simulink model "RPM_test"  (R2024a)
settings: Solver=FixedStepAuto  StartTime=0.0  StopTime=6  FixedStep=1e-5  RelTol=1e-3
values from neighbouring files (symbols this model uses):
  B = 0.002277    [initial_value.m]
  J = 0.00782    [initial_value.m]
  Lambda_m = 0.30175    [initial_value.m]
  Ld = 18e-3    (= 0.018)    [initial_value.m]
  Ldq = Ld - Lq    [inital.m]
  Lq = 32e-3    (= 0.032)    [initial_value.m]
  Polepairs = 3    [initial_value.m]
  Rs = 2.5    [initial_value.m]
  timestep = 1e-5    (= 1e-05)    [inital.m]
  V = [V_11 V_12;V_21 V_22]    [Create_MVG.m]
undefined symbols (not defined in the file or in its folder): sigbuilder_block
libraries: spsControlledVoltageSourceLib x3, spsPermanentMagnetSynchronousMachineLib x1, spsGroundLib x1, sps_lib x1
settings Model: Creator=User  LastModifiedBy=User

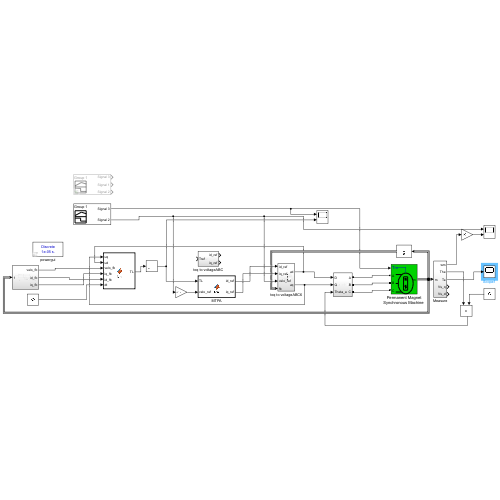
[thumbnail: Simulink's stored preview of the top-level diagram]
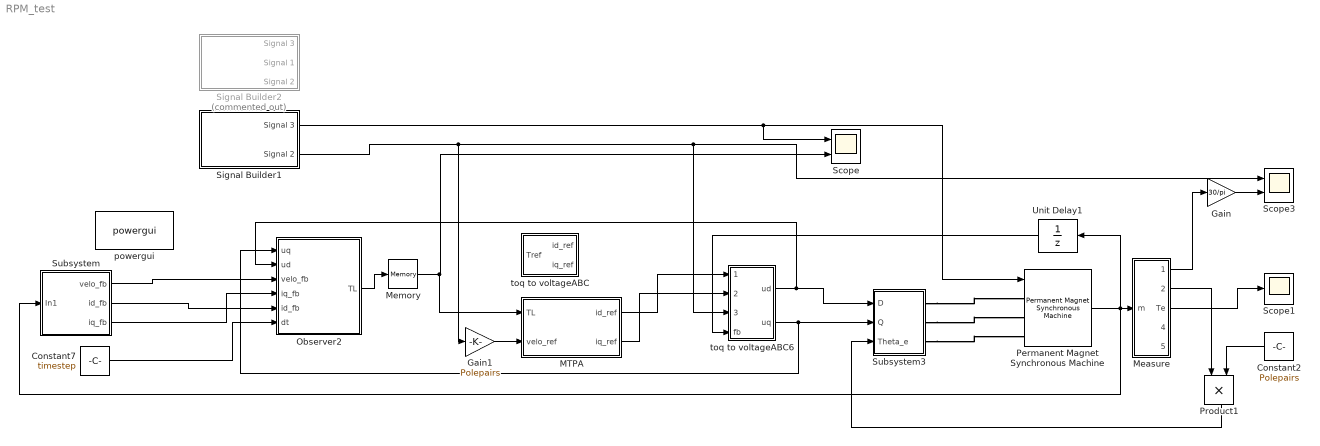
== system RPM_test ==
  Constant2 : Constant  Value=Polepairs
  Constant7 : Constant  Value=timestep
  Gain : Gain  Gain=30/pi
  Gain1 : Gain  Gain=Polepairs
  MTPA : MATLAB Function  TreatAsAtomicUnit=on
  Measure : Subsystem
  Memory : Memory
  Observer2 : MATLAB Function  TreatAsAtomicUnit=on
  "Permanent Magnet Synchronous Machine " : spsPermanentMagnetSynchronousMachineLib/Permanent Magnet Synchronous Machine  NbPhases=3  FluxDistribution=Sinusoidal  RotorType=Salient-pole  MechanicalLoad=Torque Tm  PresetModel=No  ShowDetailedParameters=on  MeasurementBus=off  Resistance=Rs  Inductance=8.5e-3  dqInductances=[Ld Lq]  La=5.7e-3  MachineConstant=Flux linkage established by magnets (V.s)  Flux=Lambda_m  VoltageCst=14.8877  TorqueCst=0.12312  Flat=120  Mechanical=[J B Polepairs]  PolePairs=4  InitialConditions=[0,0, 0,0]  InitialConditions5ph=[0 0 0 0 0 0]  RefAngle=Aligned with phase A axis (original Park)  IterativeDiscreteModel=Trapezoidal non iterative  TsBlock=-1  TsPowergui=0
  Product1 : Product
  Scope : Scope  NumInputPorts=2
  Scope1 : Scope
  Scope3 : Scope  NumInputPorts=2
  Signal Builder1 : Subsystem  Tag=STV Subsys  LoadFcn=sigbuilder_block('load');  StartFcn=sigbuilder_block('start');  StopFcn=sigbuilder_block('stop');  ClipboardFcn=sigbuilder_block('clipboard');  mask(Sigbuilder block){tuvar=[0:10]}
      mask help: Simulink:masks:SigbuilderBlock_MD
      mask init:
      | if ~strcmp(get_param(bdroot(gcbh),'SimulationStatus'),'stopped') tuvar = sigbuilder_block('maskInit'); end
      settings: CopyFcn=sigbuilder_block('copy');  DeleteFcn=sigbuilder_block('delete');  ModelCloseFcn=sigbuilder_block('modelClose');  PreSaveFcn=sigbuilder_block('preSave');  PauseFcn=sigbuilder_block('pause');  ContinueFcn=sigbuilder_block('continue');  NameChangeFcn=sigbuilder_block('namechange');  OpenFcn=sigbuilder_block('open',[524.25 120.75 551.25 399.75 ]);  CloseFcn=sigbuilder_block('close');
      mask Display: plot(0, 0, 100, 100,[2, 2, 32, 32, 2], [68, 8, 8, 68, 68],[32, 2], [38, 38], [32, 19, 2],[53, 60, 44], [32, 17, 17, 2],[16, 16, 31, 31]);txt = getActiveGroup(gcbh);text(2, 100, txt,'verticalAlignment', 'top');
  Signal Builder2 : Subsystem  Tag=STV Subsys  Commented=on  LoadFcn=sigbuilder_block('load');  StartFcn=sigbuilder_block('start');  StopFcn=sigbuilder_block('stop');  ClipboardFcn=sigbuilder_block('clipboard');  mask(Sigbuilder block){tuvar=[0:10]}
      mask help: Simulink:masks:SigbuilderBlock_MD
      mask init:
      | if ~strcmp(get_param(bdroot(gcbh),'SimulationStatus'),'stopped') tuvar = sigbuilder_block('maskInit'); end
      settings: CopyFcn=sigbuilder_block('copy');  DeleteFcn=sigbuilder_block('delete');  ModelCloseFcn=sigbuilder_block('modelClose');  PreSaveFcn=sigbuilder_block('preSave');  PauseFcn=sigbuilder_block('pause');  ContinueFcn=sigbuilder_block('continue');  NameChangeFcn=sigbuilder_block('namechange');  OpenFcn=sigbuilder_block('open',[524.25 120.75 551.25 399.75 ]);  CloseFcn=sigbuilder_block('close');
      mask Display: plot(0, 0, 100, 100,[2, 2, 32, 32, 2], [68, 8, 8, 68, 68],[32, 2], [38, 38], [32, 19, 2],[53, 60, 44], [32, 17, 17, 2],[16, 16, 31, 31]);txt = getActiveGroup(gcbh);text(2, 100, txt,'verticalAlignment', 'top');
  Subsystem : Subsystem
  Subsystem3 : Subsystem
  Unit Delay1 : UnitDelay  SampleTime=1e-5  HasFrameUpgradeWarning=on
  powergui : sps_lib/powergui  Priority=1  SimulationMode=Discrete  SampleTime=timestep  frequency=60  Iterations=50  frequencyindice=0  Pbase=100e6  ErrMax=1e-4  UnitsV=kV  UnitsW=MW  buscounter=0  FunctionMessages=off  echomessages=off  EnableUseOfTLC=off  CurrentSourceSwitches=off  DisableSnubberDevices=off  DisableRonSwitches=off  DisableVfSwitches=off  DisplayEquations=off  AutomaticDiscreteSolvers=off  SolverType=Tustin/Backward Euler (TBE)  Interpol=off  ExternalGateDelay=off  methode=off  Ts=100  x0status=blocks  SPID=on  SwTol=0  HookPort=off  NonlinearTolerance=1e-4  nMaxIteration=100  ContinueOnMaxIteration=off  RestoreLinks=warning  ResistiveCurrentMeasurement=off  Frange=[0:2:500]  Ylog=off  Xlog=on  ShowGrid=off  save=off  variable=ZData  structure=0  ZoomFFT=off  StartTime=0.0  cycles=1  DisplayStyle=1  fundamental=60  FreqAxis=off  MaxFrequency=1000  frequencyindicesteady=1  RmsSteady=1  display=off
  toq to voltageABC : Subsystem
  toq to voltageABC6 : Subsystem
  wires:
  "Permanent Magnet Synchronous Machine "/1 -> Unit Delay1/1, Measure/1(m), Subsystem/1(In1)
  Constant2/1 -> Product1/2
  Measure/2(The) -> Product1/1
  Unit Delay1/1 -> toq to voltageABC6/4(fb)
  toq to voltageABC6/1(ud) -> Observer2/2(ud), Subsystem3/1(D)
  toq to voltageABC6/2(uq) -> Observer2/1(uq), Subsystem3/2(Q)
  Product1/1 -> Subsystem3/3(Theta_e)
  Subsystem/1(velo_fb) -> Observer2/3(velo_fb)
  Subsystem/2(id_fb) -> Observer2/5(id_fb)
  Subsystem/3(iq_fb) -> Observer2/4(iq_fb)
  Signal Builder1/2(Signal 2) -> Gain1/1, toq to voltageABC6/3(velo_ref), Scope3/1
  Observer2/1(TL) -> Memory/1
  Constant7/1 -> Observer2/6(dt)
  Measure/1(wm) -> Gain/1
  Gain/1 -> Scope3/2
  Signal Builder1/1(Signal 3) -> "Permanent Magnet Synchronous Machine "/1, Scope/1
  Gain1/1 -> MTPA/2(velo_ref)
  Memory/1 -> MTPA/1(TL), Scope/2
  Measure/3(Te) -> Scope1/1
  MTPA/1(id_ref) -> toq to voltageABC6/1(id_ref)
  MTPA/2(iq_ref) -> toq to voltageABC6/2(iq_ref)
  connections:
  Subsystem3/RConn1 -- "Permanent Magnet Synchronous Machine "/LConn1
  Subsystem3/RConn2 -- "Permanent Magnet Synchronous Machine "/LConn2
  Subsystem3/RConn3 -- "Permanent Magnet Synchronous Machine "/LConn3

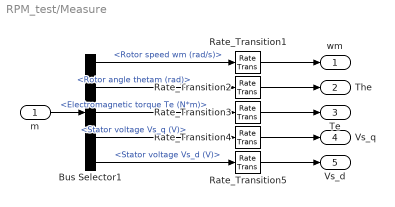
== system RPM_test/Measure ==
  m : Inport
  Bus Selector1 : BusSelector  OutputSignals=Rotor speed wm (rad/s),Rotor angle thetam (rad),Electromagnetic torque Te (N*m),Stator voltage Vs_q (V),Stator voltage Vs_d (V)
  Rate_Transition{1..5} (5 alike) : RateTransition  Integrity=off
  wm : Outport
  The : Outport  Port=2
  Te : Outport  Port=3
  Vs_q : Outport  Port=4
  Vs_d : Outport  Port=5
  wires:
  Bus Selector1/5 -> Rate_Transition5/1  "<Stator voltage Vs_d (V)>"
  Bus Selector1/4 -> Rate_Transition4/1  "<Stator voltage Vs_q (V)>"
  Bus Selector1/1 -> Rate_Transition1/1  "<Rotor speed wm (rad/s)>"
  m/1 -> Bus Selector1/1
  Bus Selector1/3 -> Rate_Transition3/1  "<Electromagnetic torque Te (N*m)>"
  Bus Selector1/2 -> Rate_Transition2/1  "<Rotor angle thetam (rad)>"
  Rate_Transition1/1 -> wm/1
  Rate_Transition2/1 -> The/1
  Rate_Transition3/1 -> Te/1
  Rate_Transition4/1 -> Vs_q/1
  Rate_Transition5/1 -> Vs_d/1

== system RPM_test/Signal Builder1 ==
  Demux : Demux  Tag=STV Demux  Outputs=2
      settings: DisplayOption=none
  FromWs : FromWorkspace  Tag=STV FromWs  VariableName=tuvar
      SigBuilderData=|
      | common.afterFinalStr = 'Extrapolate'
      | common.sampleTime = 0
      | dataSet.timeRange = [0 6]
      | dataSet.name = 'Group 1'
      | sbobj.Groups.Name = 'Group 1'
      | sbobj.Groups.Signals(1).Name = 'Signal 3'
      | sbobj.Groups.Signals(1).XData = [0 2 3 4 5 6]
      | sbobj.Groups.Signals(1).YData = [0 0 1 1 0 0]
      | sbobj.Groups.Signals(2).Name = 'Signal 2'
      | sbobj.Groups.Signals(2).XData = [0 2 3 6]
      | sbobj.Groups.Signals(2).YData = [0 10 10 10]
      | sbobj.Groups.TimeRange = [0 6]
  Signal 3 : Outport  Tag=STV Outport
  Signal 2 : Outport  Tag=STV Outport  Port=2
  wires:
  FromWs/1 -> Demux/1
  Demux/1 -> Signal 3/1
  Demux/2 -> Signal 2/1

== system RPM_test/Signal Builder2 ==
  Demux : Demux  Tag=STV Demux  Outputs=3
      settings: DisplayOption=none
  FromWs : FromWorkspace  Tag=STV FromWs  VariableName=tuvar
      SigBuilderData=|
      | common.afterFinalStr = 'Extrapolate'
      | common.sampleTime = 0
      | dataSet.timeRange = [0 6]
      | dataSet.name = 'Group 1'
      | sbobj.Groups.Name = 'Group 1'
      | sbobj.Groups.Signals(1).Name = 'Signal 3'
      | sbobj.Groups.Signals(1).XData = [0 6]
      | sbobj.Groups.Signals(1).YData = [1 1]
      | sbobj.Groups.Signals(2).Name = 'Signal 1'
      | sbobj.Groups.Signals(2).XData = [0 2 4 6]
      | sbobj.Groups.Signals(2).YData = [0 1.5 1.5 0]
      | sbobj.Groups.Signals(3).Name = 'Signal 2'
      | sbobj.Groups.Signals(3).XData = [0 6]
      | sbobj.Groups.Signals(3).YData = [0 10]
      | sbobj.Groups.TimeRange = [0 6]
  Signal 3 : Outport  Tag=STV Outport
  Signal 1 : Outport  Tag=STV Outport  Port=2
  Signal 2 : Outport  Tag=STV Outport  Port=3
  wires:
  FromWs/1 -> Demux/1
  Demux/1 -> Signal 3/1
  Demux/2 -> Signal 1/1
  Demux/3 -> Signal 2/1

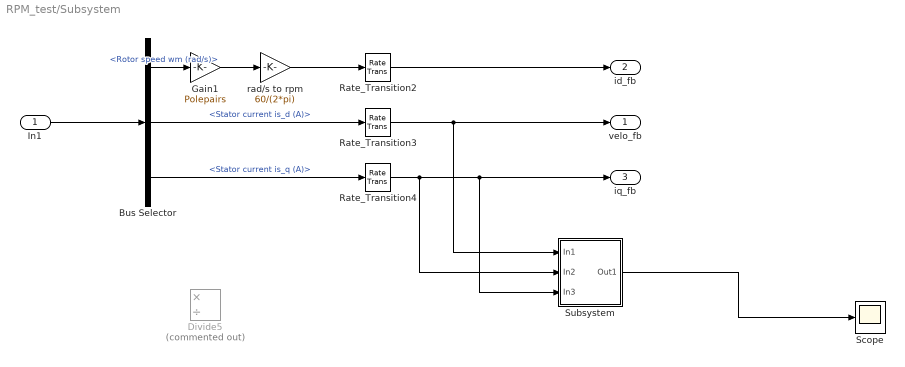
== system RPM_test/Subsystem ==
  In1 : Inport
  Bus Selector : BusSelector  OutputSignals=Rotor speed wm (rad/s),Stator current is_d (A),Stator current is_q (A)
  Divide5 : Product  Commented=on  Inputs=*/
  Gain1 : Gain  Gain=Polepairs
  Rate_Transition2 : RateTransition  Integrity=off  Deterministic=off
  Rate_Transition3 : RateTransition  Integrity=off  Deterministic=off
  Rate_Transition4 : RateTransition  Integrity=off  Deterministic=off
  Scope : Scope
  Subsystem : Subsystem
  rad/s to rpm : Gain  Gain=60/(2*pi)
  velo_fb : Outport
  id_fb : Outport  Port=2
  iq_fb : Outport  Port=3
  wires:
  Gain1/1 -> rad/s to rpm/1
  rad/s to rpm/1 -> Rate_Transition2/1
  Rate_Transition4/1 -> Subsystem/2(In2), Subsystem/3(In3), iq_fb/1
  Bus Selector/1 -> Gain1/1  "<Rotor speed wm (rad/s)>"
  Bus Selector/3 -> Rate_Transition4/1  "<Stator current is_q (A)>"
  Bus Selector/2 -> Rate_Transition3/1  "<Stator current is_d (A)>"
  In1/1 -> Bus Selector/1
  Rate_Transition3/1 -> Subsystem/1(In1), velo_fb/1
  Rate_Transition2/1 -> id_fb/1
  Subsystem/1(Out1) -> Scope/1

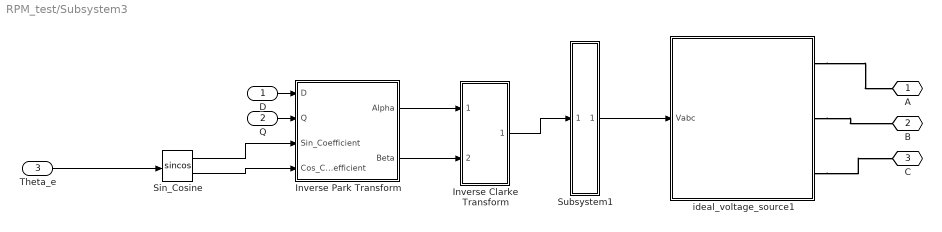
== system RPM_test/Subsystem3 ==
  D : Inport
  Q : Inport  Port=2
  Theta_e : Inport  Port=3
  Inverse Clarke Transform : Subsystem
  Inverse Park Transform : Subsystem
  Sin_Cosine : Trigonometry  Operator=sincos
  Subsystem1 : Subsystem
      mask Display: fprintf('D/C')
  ideal_voltage_source1 : Subsystem  VariantControl=variantPwm == enumPwm.behavior
  A : PMIOPort  Side=Right
  B : PMIOPort  Port=2  Side=Right
  C : PMIOPort  Port=3  Side=Right
  wires:
  D/1 -> Inverse Park Transform/1(D)
  Inverse Park Transform/1(Alpha) -> Inverse Clarke Transform/1(Alpha)
  Sin_Cosine/1 -> Inverse Park Transform/3(Sin_Coefficient)
  Theta_e/1 -> Sin_Cosine/1
  Sin_Cosine/2 -> Inverse Park Transform/4(Cos_Coefficient)
  Inverse Park Transform/2(Beta) -> Inverse Clarke Transform/2(Beta)
  Subsystem1/1(Out1) -> ideal_voltage_source1/1(Vabc)
  Inverse Clarke Transform/1(ABC) -> Subsystem1/1(In1)
  Q/1 -> Inverse Park Transform/2(Q)
  connections:
  ideal_voltage_source1/RConn2 -- B/RConn1
  ideal_voltage_source1/RConn3 -- C/RConn1
  ideal_voltage_source1/RConn1 -- A/RConn1

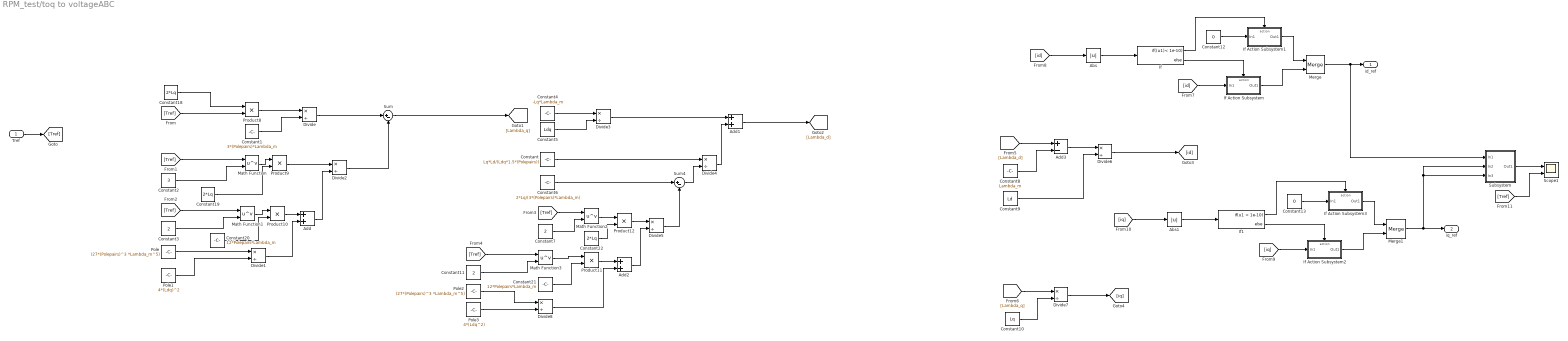
== system RPM_test/toq to voltageABC ==
  Tref : Inport
  Abs : Abs  SaturateOnIntegerOverflow=off
  Abs1 : Abs  SaturateOnIntegerOverflow=off
  Add : Sum
  Add1 : Sum
  Add2 : Sum
  Add3 : Sum  Inputs=+-
  Constant : Constant  Value=Lq*Ld/(Ldq*1.5*(Polepairs))
  Constant1 : Constant  Value=3*(Polepairs)*Lambda_m
  Constant10 : Constant  Value=Lq
  Constant11 : Constant  Value=2
  Constant12 : Constant  Value=0
  Constant13 : Constant  Value=0
  Constant18 : Constant  Value=2*Lq
  Constant19 : Constant  Value=2*Lq
  Constant2 : Constant  Value=3
  Constant20 : Constant  Value=12*Polepairs*Lambda_m
  Constant21 : Constant  Value=12*Polepairs*Lambda_m
  Constant22 : Constant  Value=2*Lq
  Constant3 : Constant  Value=2
  Constant4 : Constant  Value=-Lq*Lambda_m
  Constant5 : Constant  Value=Ldq
  Constant6 : Constant  Value=2*Lq/(3*(Polepairs)*Lambda_m)
  Constant7 : Constant  Value=2
  Constant8 : Constant  Value=Lambda_m
  Constant9 : Constant  Value=Ld
  Divide{,1..8} (9 alike) : Product  Inputs=*/
  If : If  IfExpression=(u1)< 1e-10
  If Action Subsystem : Subsystem  TreatAsAtomicUnit=on
  If Action Subsystem1 : Subsystem  TreatAsAtomicUnit=on
  If Action Subsystem2 : Subsystem  TreatAsAtomicUnit=on
  If Action Subsystem3 : Subsystem  TreatAsAtomicUnit=on
  If1 : If  IfExpression=u1 < 1e-10
  Math Function{,1..3} (4 alike) : Math  Operator=pow
  Merge : Merge
  Merge1 : Merge
  Pole : Constant  Value=(27*(Polepairs)^3 *Lambda_m^5)
  Pole1 : Constant  Value=4*(Ldq)^2
  Pole2 : Constant  Value=(27*(Polepairs)^3 *Lambda_m^5)
  Pole3 : Constant  Value=4*(Ldq^2)
  Product{8..12} (5 alike) : Product
  Scope1 : Scope  NumInputPorts=2
  Subsystem : Subsystem
  Sum : Sum  Inputs=|+-
  Sum4 : Sum  Inputs=|+-
  id_ref : Outport
  iq_ref : Outport  Port=2
  wires:
  Tref/1 -> [Tref]
  [Tref] -> Product8/2
  Product8/1 -> Divide/1
  Constant1/1 -> Divide/2
  [Tref] -> Math Function/1
  Constant2/1 -> Math Function/2
  [Tref] -> Math Function1/1
  Constant3/1 -> Math Function1/2
  Product10/1 -> Add/1
  Pole/1 -> Divide1/1
  Pole1/1 -> Divide1/2
  Divide1/1 -> Add/2
  Add/1 -> Divide2/2
  Product9/1 -> Divide2/1
  Divide/1 -> Sum/1
  Divide2/1 -> Sum/2
  Constant18/1 -> Product8/1
  Math Function/1 -> Product9/1
  Constant19/1 -> Product9/2
  Math Function1/1 -> Product10/1
  Constant20/1 -> Product10/2
  Sum/1 -> [Lambda_q]
  [Lambda_d] -> Add3/1
  Constant8/1 -> Add3/2
  Add3/1 -> Divide6/1
  Constant9/1 -> Divide6/2
  Divide6/1 -> [id]
  [Lambda_q] -> Divide7/1
  Constant10/1 -> Divide7/2
  Pole2/1 -> Divide8/1
  Constant7/1 -> Math Function2/2
  Add1/1 -> [Lambda_d]
  Divide3/1 -> Add1/1
  Constant4/1 -> Divide3/1
  Product12/1 -> Divide5/1
  Constant22/1 -> Product12/2
  Constant21/1 -> Product11/2
  Math Function3/1 -> Product11/1
  Math Function2/1 -> Product12/1
  Product11/1 -> Add2/1
  Constant/1 -> Divide4/1
  [Tref] -> Math Function2/1
  Divide4/1 -> Add1/2
  Sum4/1 -> Divide4/2
  Constant11/1 -> Math Function3/2
  Constant6/1 -> Sum4/1
  Pole3/1 -> Divide8/2
  Add2/1 -> Divide5/2
  Divide8/1 -> Add2/2
  [Tref] -> Math Function3/1
  Constant5/1 -> Divide3/2
  Divide5/1 -> Sum4/2
  If/2 -> If Action Subsystem/Action
  If/1 -> If Action Subsystem1/Action
  Constant12/1 -> If Action Subsystem1/1(In1)
  If Action Subsystem1/1(Out1) -> Merge/1
  If Action Subsystem/1(Out1) -> Merge/2
  Merge/1 -> Subsystem/1(In1), id_ref/1
  [id] -> If Action Subsystem/1(In1)
  Divide7/1 -> [iq]
  [id] -> Abs/1
  If Action Subsystem2/1(Out1) -> Merge1/2
  [iq] -> If Action Subsystem2/1(In1)
  If Action Subsystem3/1(Out1) -> Merge1/1
  If1/2 -> If Action Subsystem2/Action
  Merge1/1 -> Subsystem/3(In3), Subsystem/2(In2), iq_ref/1
  If1/1 -> If Action Subsystem3/Action
  Constant13/1 -> If Action Subsystem3/1(In1)
  [iq] -> Abs1/1
  Abs/1 -> If/1
  Abs1/1 -> If1/1
  Subsystem/1(Out1) -> Scope1/1
  [Tref] -> Scope1/2

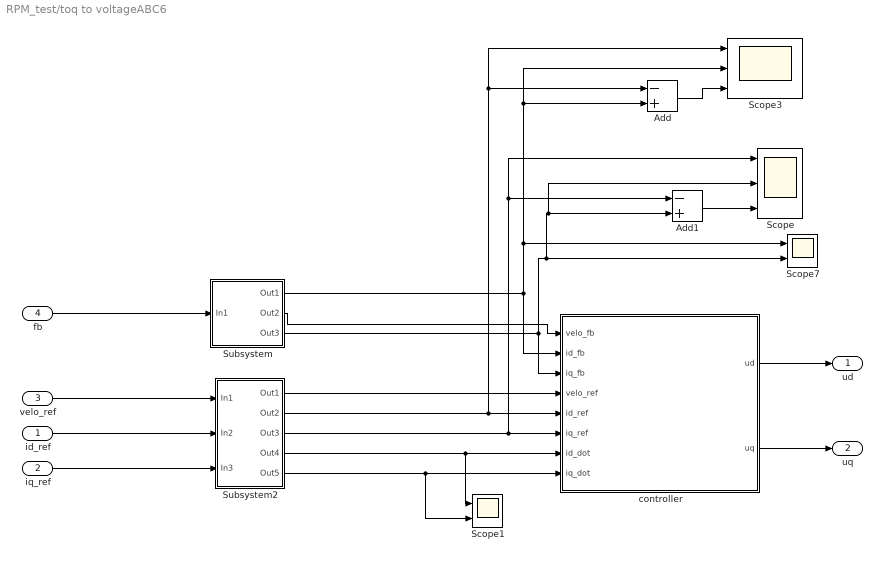
== system RPM_test/toq to voltageABC6 ==
  id_ref : Inport
  iq_ref : Inport  Port=2
  velo_ref : Inport  Port=3
  fb : Inport  Port=4
  Add : Sum  Inputs=-+
  Add1 : Sum  Inputs=-+
  Scope : Scope  NumInputPorts=3
  Scope1 : Scope  NumInputPorts=2
  Scope3 : Scope  NumInputPorts=3
  Scope7 : Scope  NumInputPorts=2
  Subsystem : Subsystem
  Subsystem2 : Subsystem
  controller : MATLAB Function  TreatAsAtomicUnit=on
  ud : Outport
  uq : Outport  Port=2
  wires:
  Add/1 -> Scope3/3
  Add1/1 -> Scope/3
  Subsystem/3(Out3) -> controller/3(iq_fb), Scope7/2, Scope/2, Add1/2
  Subsystem/2(Out2) -> controller/1(velo_fb)
  Subsystem/1(Out1) -> Scope7/1, Scope3/2, Add/2, controller/2(id_fb)
  fb/1 -> Subsystem/1(In1)
  Subsystem2/3(Out3) -> Scope/1, Add1/1, controller/6(iq_ref)
  Subsystem2/2(Out2) -> Scope3/1, Add/1, controller/5(id_ref)
  Subsystem2/1(Out1) -> controller/4(velo_ref)
  Subsystem2/4(Out4) -> Scope1/1, controller/7(id_dot)
  Subsystem2/5(Out5) -> Scope1/2, controller/8(iq_dot)
  velo_ref/1 -> Subsystem2/1(In1)
  id_ref/1 -> Subsystem2/2(In2)
  iq_ref/1 -> Subsystem2/3(In3)
  controller/1(ud) -> ud/1
  controller/2(uq) -> uq/1

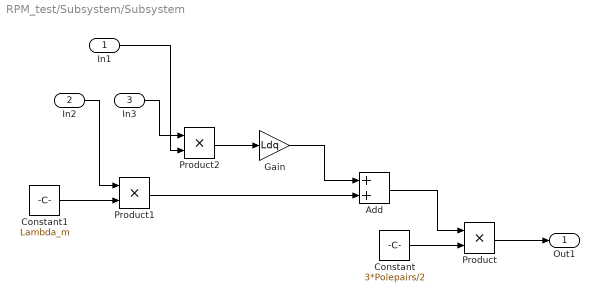
== system RPM_test/Subsystem/Subsystem ==
  In1 : Inport
  In2 : Inport  Port=2
  In3 : Inport  Port=3
  Add : Sum
  Constant : Constant  Value=3*Polepairs/2
  Constant1 : Constant  Value=Lambda_m
  Gain : Gain  Gain=Ldq
  Product : Product
  Product1 : Product
  Product2 : Product
  Out1 : Outport
  wires:
  Product1/1 -> Add/2
  Product2/1 -> Gain/1
  Product/1 -> Out1/1
  Constant/1 -> Product/2
  In3/1 -> Product2/1
  Add/1 -> Product/1
  Gain/1 -> Add/1
  Constant1/1 -> Product1/2
  In1/1 -> Product2/2
  In2/1 -> Product1/1

== system RPM_test/Subsystem3/Inverse Clarke Transform ==
  note: Inverse Clarke Transform
  note: Converts direct axis (alpha) component and the quadrature axis (beta) component to balanced three-phase quantities
      | The alpha and beta components are dependent on time and speed.
  Alpha : Inport
  Beta : Inport  Port=2
  Add : Sum  Inputs=-+  OutDataTypeStr=Inherit: Same as first input
  Add1 : Sum  Inputs=--  OutDataTypeStr=Inherit: Same as first input
  Gain : Gain  Gain=1/2
  Gain1 : Gain  Gain=sqrt(3)/2
  Mux : Mux  Inputs=3
  ABC : Outport  VectorParamsAs1DForOutWhenUnconnected=off
  wires:
  Beta/1 -> Gain1/1
  Mux/1 -> ABC/1
  Alpha/1 -> Mux/1, Gain/1
  Add1/1 -> Mux/3
  Gain1/1 -> Add1/2, Add/2
  Gain/1 -> Add1/1, Add/1
  Add/1 -> Mux/2

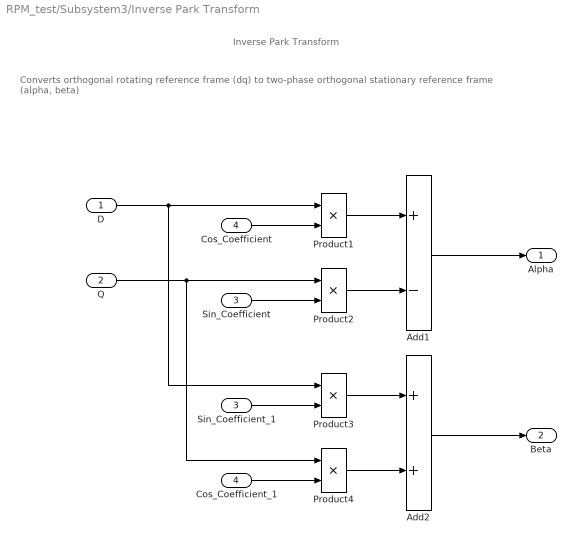
== system RPM_test/Subsystem3/Inverse Park Transform ==
  note: Converts orthogonal rotating reference frame (dq) to two-phase orthogonal stationary reference frame (alpha, beta)
  note: Inverse Park Transform
  D : Inport
  Q : Inport  Port=2
  Sin_Coefficient : Inport  Port=3
  Cos_Coefficient : Inport  Port=4
  Add1 : Sum  Inputs=+-  OutDataTypeStr=Inherit: Same as first input
  Add2 : Sum  OutDataTypeStr=Inherit: Same as first input
  Cos_Coefficient_1 : InportShadow  Port=4
  Product{1..4} (4 alike) : Product  RndMeth=Simplest
  Sin_Coefficient_1 : InportShadow  Port=3
  Alpha : Outport  VectorParamsAs1DForOutWhenUnconnected=off
  Beta : Outport  Port=2  VectorParamsAs1DForOutWhenUnconnected=off
  wires:
  Sin_Coefficient_1/1 -> Product3/2
  Product2/1 -> Add1/2
  Cos_Coefficient_1/1 -> Product4/2
  Add2/1 -> Beta/1
  Product3/1 -> Add2/1
  Add1/1 -> Alpha/1
  Product1/1 -> Add1/1
  Product4/1 -> Add2/2
  Sin_Coefficient/1 -> Product2/2
  D/1 -> Product3/1, Product1/1
  Q/1 -> Product2/1, Product4/1
  Cos_Coefficient/1 -> Product1/2

== system RPM_test/Subsystem3/Subsystem1 ==
  In1 : Inport
  Rate_Transition1 : RateTransition  Integrity=off
  Out1 : Outport  VectorParamsAs1DForOutWhenUnconnected=off
  wires:
  In1/1 -> Rate_Transition1/1
  Rate_Transition1/1 -> Out1/1

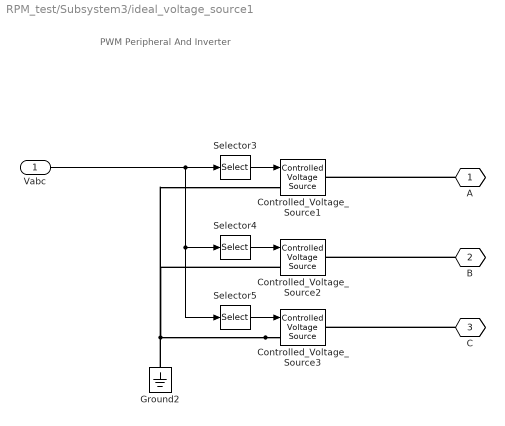
== system RPM_test/Subsystem3/ideal_voltage_source1 ==
  note: PWM Peripheral And Inverter
  Vabc : Inport
  Controlled_Voltage_Source1 : spsControlledVoltageSourceLib/Controlled Voltage Source  Initialize=off  Source_Type=DC  Amplitude=12  Phase=0  Frequency=0  Measurements=None
  Controlled_Voltage_Source2 : spsControlledVoltageSourceLib/Controlled Voltage Source  Initialize=off  Source_Type=DC  Amplitude=12  Phase=0  Frequency=0  Measurements=None
  Controlled_Voltage_Source3 : spsControlledVoltageSourceLib/Controlled Voltage Source  Initialize=off  Source_Type=DC  Amplitude=12  Phase=0  Frequency=0  Measurements=None
  Ground2 : spsGroundLib/Ground  LConnTagsString=a
  Selector3 : Selector  InputPortWidth=3  IndexOptions=Index vector (dialog)  Indices=[1]  OutputSizes=1
  Selector4 : Selector  InputPortWidth=3  IndexOptions=Index vector (dialog)  Indices=2  OutputSizes=1
  Selector5 : Selector  InputPortWidth=3  IndexOptions=Index vector (dialog)  Indices=3  OutputSizes=1
  A : PMIOPort  Tag=PMCPort  Side=Right
  B : PMIOPort  Tag=PMCPort  Port=2  Side=Right
  C : PMIOPort  Tag=PMCPort  Port=3  Side=Right
  wires:
  Vabc/1 -> Selector4/1, Selector5/1, Selector3/1
  Selector5/1 -> Controlled_Voltage_Source3/1
  Selector4/1 -> Controlled_Voltage_Source2/1
  Selector3/1 -> Controlled_Voltage_Source1/1
  connections:
  C/RConn1 -- Controlled_Voltage_Source3/RConn1
  B/RConn1 -- Controlled_Voltage_Source2/RConn1
  A/RConn1 -- Controlled_Voltage_Source1/RConn1
  Controlled_Voltage_Source3/LConn1 -- Controlled_Voltage_Source1/LConn1 -- Controlled_Voltage_Source2/LConn1 -- Ground2/LConn1

== system RPM_test/toq to voltageABC/If Action Subsystem ==
  In1 : Inport
  Action Port : ActionPort  ActionPortLabel=else
  Out1 : Outport
  wires:
  In1/1 -> Out1/1

== system RPM_test/toq to voltageABC/If Action Subsystem1 ==
  In1 : Inport
  Action Port : ActionPort  ActionPortLabel=if((u1)< 1e-10)
  Out1 : Outport
  wires:
  In1/1 -> Out1/1

== system RPM_test/toq to voltageABC/If Action Subsystem2 ==
  In1 : Inport
  Action Port : ActionPort  ActionPortLabel=else
  Out1 : Outport
  wires:
  In1/1 -> Out1/1

== system RPM_test/toq to voltageABC/If Action Subsystem3 ==
  In1 : Inport
  Action Port : ActionPort  ActionPortLabel=if(u1 < 1e-10)
  Out1 : Outport
  wires:
  In1/1 -> Out1/1

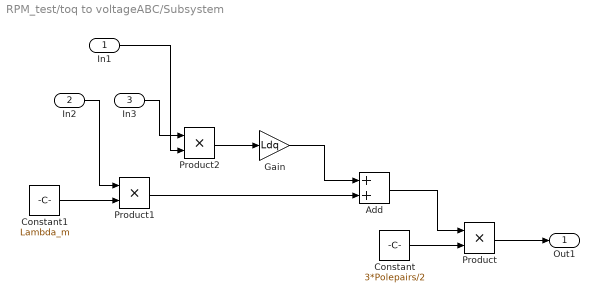
== system RPM_test/toq to voltageABC/Subsystem ==
  In1 : Inport
  In2 : Inport  Port=2
  In3 : Inport  Port=3
  Add : Sum
  Constant : Constant  Value=3*Polepairs/2
  Constant1 : Constant  Value=Lambda_m
  Gain : Gain  Gain=Ldq
  Product : Product
  Product1 : Product
  Product2 : Product
  Out1 : Outport
  wires:
  Product1/1 -> Add/2
  Product2/1 -> Gain/1
  Product/1 -> Out1/1
  Constant/1 -> Product/2
  In3/1 -> Product2/1
  Add/1 -> Product/1
  Gain/1 -> Add/1
  Constant1/1 -> Product1/2
  In1/1 -> Product2/2
  In2/1 -> Product1/1

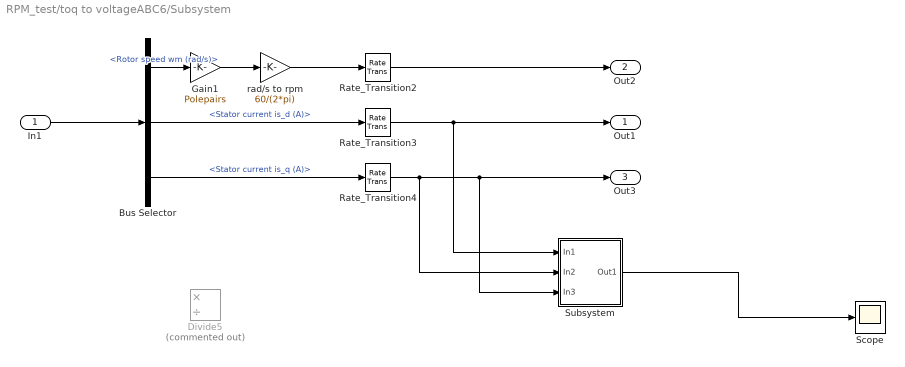
== system RPM_test/toq to voltageABC6/Subsystem ==
  In1 : Inport
  Bus Selector : BusSelector  OutputSignals=Rotor speed wm (rad/s),Stator current is_d (A),Stator current is_q (A)
  Divide5 : Product  Commented=on  Inputs=*/
  Gain1 : Gain  Gain=Polepairs
  Rate_Transition2 : RateTransition  Integrity=off  Deterministic=off
  Rate_Transition3 : RateTransition  Integrity=off  Deterministic=off
  Rate_Transition4 : RateTransition  Integrity=off  Deterministic=off
  Scope : Scope
  Subsystem : Subsystem
  rad/s to rpm : Gain  Gain=60/(2*pi)
  Out1 : Outport
  Out2 : Outport  Port=2
  Out3 : Outport  Port=3
  wires:
  Rate_Transition4/1 -> Subsystem/2(In2), Subsystem/3(In3), Out3/1
  Bus Selector/1 -> Gain1/1  "<Rotor speed wm (rad/s)>"
  Bus Selector/3 -> Rate_Transition4/1  "<Stator current is_q (A)>"
  Bus Selector/2 -> Rate_Transition3/1  "<Stator current is_d (A)>"
  In1/1 -> Bus Selector/1
  Rate_Transition3/1 -> Subsystem/1(In1), Out1/1
  Rate_Transition2/1 -> Out2/1
  Subsystem/1(Out1) -> Scope/1
  Gain1/1 -> rad/s to rpm/1
  rad/s to rpm/1 -> Rate_Transition2/1

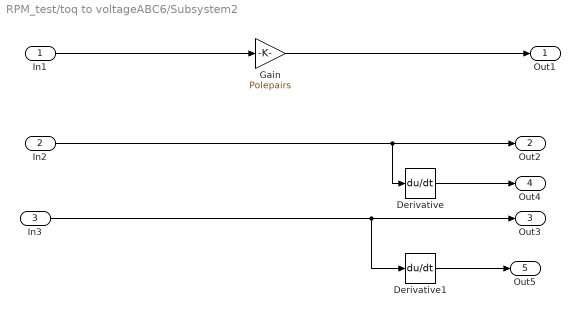
== system RPM_test/toq to voltageABC6/Subsystem2 ==
  In1 : Inport
  In2 : Inport  Port=2
  In3 : Inport  Port=3
  Derivative : Derivative
  Derivative1 : Derivative
  Gain : Gain  Gain=Polepairs
  Out1 : Outport
  Out2 : Outport  Port=2
  Out3 : Outport  Port=3
  Out4 : Outport  Port=4
  Out5 : Outport  Port=5
  wires:
  In2/1 -> Derivative/1, Out2/1
  In1/1 -> Gain/1
  In3/1 -> Derivative1/1, Out3/1
  Derivative/1 -> Out4/1
  Derivative1/1 -> Out5/1
  Gain/1 -> Out1/1

== system RPM_test/toq to voltageABC6/Subsystem/Subsystem ==
  In1 : Inport
  In2 : Inport  Port=2
  In3 : Inport  Port=3
  Add : Sum
  Constant : Constant  Value=3*Polepairs/2
  Constant1 : Constant  Value=Lambda_m
  Gain : Gain  Gain=Ldq
  Product : Product
  Product1 : Product
  Product2 : Product
  Out1 : Outport
  wires:
  Product1/1 -> Add/2
  Product2/1 -> Gain/1
  Product/1 -> Out1/1
  Constant/1 -> Product/2
  In3/1 -> Product2/1
  Add/1 -> Product/1
  Gain/1 -> Add/1
  Constant1/1 -> Product1/2
  In1/1 -> Product2/2
  In2/1 -> Product1/1

== matlab function RPM_test/Observer2 ==
  data: TL output; uq input; ud input; velo_fb input; iq_fb input; id_fb input; dt input
function TL = fcn(uq, ud, velo_fb, iq_fb, id_fb,dt)
    
    % 定義持久變量 x
    persistent x
    
    % 初始化 x，如果 x 是空的
    if isempty(x)
        x = zeros(4,1, 'double');  % 初始化為 4x1 向量
    end
    
    % 如果 uq 為空，設置 uq 和 ud 為 0
    if isempty(uq)
        ud = 0;
        uq = 0;
    end

    % 定義參數
    [Ld, Lq, Rs, Lambda_m, Polepairs, J, B] = initial_value();  % 初始值函數
    Ldq = Ld - Lq;


    % 輸入測量的狀態變數
    y = [velo_fb; iq_fb; id_fb];

    % 定義系統係數
    k1 = 3 * Polepairs^2 * Lambda_m / (2 * J);
    k2 = B / J;
    k3 = Polepairs / (J);
    k4 = Rs / Lq;
    k5 = Lambda_m / Lq;
    k6 = 1 / Lq;
    k7 = Rs / Ld;
    k8 = 1 / Ld;
    k9 = Lq / Ld;
    k10 = Ld / Lq;
    k11 = 3 * Polepairs^2 * Ldq / (2 * J);

    % 控制輸入 u
    u = [0; 0; k6 * uq; k8 * ud];

    % 定義系統矩陣 A_o
    A_o = [0, 0, 0, 0;
          -k3, -k2, k1, k11 * iq_fb;
           0, -k5 - k10 * id_fb, -k4, 0;
           0, k9 * iq_fb, 0, -k7];

    % 定義輸出矩陣 C_o
    C_o = [0, 1, 0, 0;
           0, 0, 1, 0;
           0, 0, 0, 1];

    % 定義權重矩陣 Q 和 R
    Q = diag([100, 100, 100, 100]);
    R = diag([1, 1, 1]);

    % 使用 SDA_CARE 求解 P_ss_care
    [P_ss_care, ~] = SDA_CARE(A_o', C_o', Q, R);

    % 計算觀察器增益 M
    M = P_ss_care * C_o' * inv(R);

    % 計算狀態變化率 x_dot
    x_dot = A_o * x + M * y - M * C_o * x + u;

    % 用積分的方法更新狀態 x
    x = x + x_dot * dt;
    

    TL = x(1);

end

== matlab function RPM_test/toq to voltageABC6/controller ==
  data: velo_fb input; id_fb input; iq_fb input; velo_ref input; id_ref input; iq_ref input; ud output; uq output; id_dot input; iq_dot input
function [ud,uq] = SDRE_motor(velo_fb,id_fb,iq_fb,velo_ref,id_ref,iq_ref,id_dot,iq_dot)

ud = zeros(1, 1, 'double');
uq = zeros(1, 1, 'double');

%change data from [1*1] to singal input
Q = zeros(3, 3, 'double');

if isempty(id_dot)
    id_dot=0;
    iq_dot=0;
end


% velo_error   = 0;
% id_error     = 0;
% iq_error     = 0;

velo_error   = velo_fb   - velo_ref;
id_error     = id_fb     - id_ref;
iq_error     = iq_fb     - iq_ref;

if isempty(iq_error)
    velo_error=0;
    id_error=0;
    iq_error =0;
end

error = [velo_error iq_error id_error];

[Ld,Lq,Rs,Lambda_m,Polepairs,J,B]  = initial_value;
Ldq = Ld-Lq;

% A11 = -B/J; A12 = 3*Polepairs^2 *Lambda_m/(8*J); A13 = 3*Polepairs^2 *Ldq*iq_error/(8*J);
% A21 = -Lambda_m/(Lq) - Ld*id_error/(2*Lq); A22 = -Rs/Lq; A23 = - Ld*velo_error/(2*Lq);
% A31 = Lq*iq_error/(2*Ld); A32 =Lq*velo_error/(2*Ld); A33 = -Rs/Ld;

A11 = -B/J; A12 = 3*Polepairs^2 *Lambda_m/(2*J); A13 = 3*Polepairs^2 *Ldq*iq_error/(2*J);
A21 = -Lambda_m/(Lq) - Ld*id_error/(Lq); A22 = -Rs/Lq; A23 = 0;
A31 = Lq*iq_error/(Ld); A32 =0; A33 = -Rs/Ld;

B11 = 0;B12 =0;
B21=1/Lq;B22=0;
B31=0;B32=1/Ld;


A = [A11 A12 A13 ;
     A21 A22 A23 ;
     A31 A32 A33];

B = [B11 B12;
     B21 B22;
     B31 B32];


rate = sqrt(iq_error^2 + id_error^2);

Q=diag([800 1+exp(-rate) 100+exp(-rate)]);
R=diag([1 1]);

[P_ss_care,~]=SDA_CARE(A,B,Q,R);


% ucq = Rs*iq_ref + Lq*iq_dot + velo_ref*(Ld*id_ref+Lambda_m);
% ucd = Rs*id_ref + Ld*id_dot - velo_ref*Lq*iq_ref;


ucq = Rs*iq_ref + Lambda_m*velo_ref + Lq*iq_dot + Ld*id_error*velo_ref + Ld*velo_fb*id_ref;
ucd = Rs*id_ref + Ld*id_dot - Lq*iq_error*velo_ref - Lq*velo_fb*iq_ref;
if ucq > 1e5
    ucq =0;
end

if ucd > 1e5
    ucd =0;
end

u_redeem = -inv(R)*B'*P_ss_care*error';

% uq =  ucq ;
% ud =  ucd ;

uq =  ucq + u_redeem(1) ;
ud =  ucd + u_redeem(2) ;

ud1 = ucd ;
uq1 = ucq;

ud2 = u_redeem(2) ;
uq2 = u_redeem(1) ;


ud = (reshape(ud, 1, 1));
uq = (reshape(uq, 1, 1));


end

== matlab function RPM_test/MTPA ==
  data: id_ref output; TL input; iq_ref output; velo_ref input
function [id_ref , iq_ref] = fcn(TL,velo_ref)

[Ld,Lq,Rs,Lambda_m,Polepairs,J,B]  = initial_value;
Ldq = Ld-Lq;

k1 = 3*Polepairs^2 *Lambda_m/(2*J);
k2 = B/J;
k3 = Polepairs/(J);
k11 = 3*Polepairs^2 *Ldq/(2*J);

p1 = Ldq*k11/Lambda_m;
p2=0;
p3 = k1;
p4 = -(k2*velo_ref+k3*TL);
p = [p1 p2 p3 p4];
r = roots(p);

real_solutions = r(imag(r) == 0);


iq_ref = real(max(real_solutions));
id_ref = Ldq*iq_ref^2 /Lambda_m;
end
